simulink model "fundamental_component_calc"  (R2023a)
settings: Solver=VariableStepAuto  StartTime=0.0  StopTime=30  RelTol=1e-3
InitFcn:
  | Ts=100e-6;
libraries: powerlib_extras x2, simulink x1
settings Model: Creator=anony  LastModifiedBy=ym
settings SolverCC: AlgebraicLoopSolver=TrustRegion
settings OptimizationCC: ReuseModelBlockBuffer=off
settings DebuggingCC: UnconnectedInputMsg=warning  UnconnectedOutputMsg=warning  UnconnectedLineMsg=warning
settings ModelReferenceCC: EnableRefExpFcnMdlSchedulingChecks=on
settings RTWCC: DLArmComputeVersion=19.05

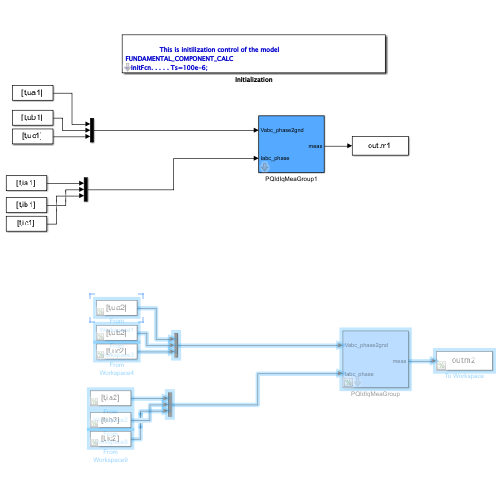
[thumbnail: Simulink's stored preview of the top-level diagram]
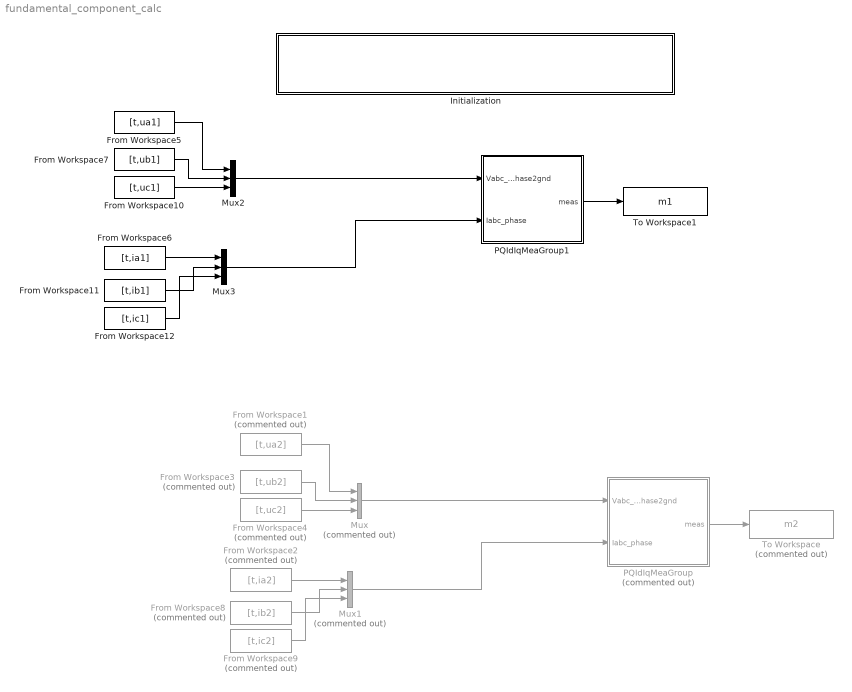
== system fundamental_component_calc ==
  From Workspace1 : FromWorkspace  Commented=on  VariableName=[t,ua2]
  From Workspace10 : FromWorkspace  VariableName=[t,uc1]
  From Workspace11 : FromWorkspace  VariableName=[t,ib1]
  From Workspace12 : FromWorkspace  VariableName=[t,ic1]
  From Workspace2 : FromWorkspace  Commented=on  VariableName=[t,ia2]
  From Workspace3 : FromWorkspace  Commented=on  VariableName=[t,ub2]
  From Workspace4 : FromWorkspace  Commented=on  VariableName=[t,uc2]
  From Workspace5 : FromWorkspace  VariableName=[t,ua1]
  From Workspace6 : FromWorkspace  VariableName=[t,ia1]
  From Workspace7 : FromWorkspace  VariableName=[t,ub1]
  From Workspace8 : FromWorkspace  Commented=on  VariableName=[t,ib2]
  From Workspace9 : FromWorkspace  Commented=on  VariableName=[t,ic2]
  Initialization : Subsystem  mask(Model Functions){InitFcnX=Ts=100e-6;, prel=off, posl=off, inif=on, strf=off}
      mask prompts: InitFcnX "Initialisation"; prel "Preload Function"; posl "PostLoad Function"; inif "InitFcn"; strf "StartFcn"
      mask init:
      | if prel==1
      | 	set_param(bdroot, 'PreLoadFcn', InitFcnX);
      | else
      | 	set_param(bdroot, 'PreLoadFcn', '');
      | end
      | if inif==1
      | 	set_param(bdroot, 'InitFcn', InitFcnX);
      | else
      | 	set_param(bdroot, 'InitFcn', '');
      | end
      | if strf==1
      | 	set_param(bdroot, 'StartFcn', InitFcnX);
      | else
      | 	set_param(bdroot, 'StartFcn', '');
      | end
      | if posl==1
      | 	set_param(bdroot, 'PostLoadFcn', InitFcnX);
      | else
      | 	set_param(bdroot, 'PostLoadFcn', '');
      | end
      | PLF = get_param(bdroot, 'PreLoadFcn');
      | IF = get_param(bdroot, 'InitFcn');
      | SF = get_param(bdroot, 'StartFcn');
      | 
      | 
      | pos = get_param(gcb, 'Position');
      | width = pos(3) - pos(1); height = pos(4) - pos(2);
      mask Display:
      | color('blue')
      | text(5, height*0.25, [ ...
      | upper(bdroot) '\n' ...
      | '- InitFcn. . . . . '  get_param(bdroot, 'InitFcn')  ...
      | ], ...
      | 'horizontalAlignment', 'left', 'verticalAlignment', 'middle') ;
      | text(60,height*0.6,'This is initilization control of the model');
  Mux : Mux  Commented=on  Inputs=3
  Mux1 : Mux  Commented=on  Inputs=3
  Mux2 : Mux  Inputs=3
  Mux3 : Mux  Inputs=3
  PQIdIqMeaGroup : Subsystem  Commented=on  mask{var_pnom=1.5e6, var_vline_rms=690, var_ts=Ts}
      mask prompts: var_pnom "Pnom"; var_vline_rms "Line voltage rms"; var_ts "Sample Time"
  PQIdIqMeaGroup1 : Subsystem  mask{var_pnom=1.5e6, var_vline_rms=690, var_ts=Ts}
      mask prompts: var_pnom "Pnom"; var_vline_rms "Line voltage rms"; var_ts "Sample Time"
  To Workspace : ToWorkspace  Commented=on  VariableName=m2  SaveFormat=Structure With Time  SampleTime=-1
  To Workspace1 : ToWorkspace  VariableName=m1  SaveFormat=Structure With Time  SampleTime=-1
  wires:
  Mux1/1 -> PQIdIqMeaGroup/2(Iabc_phase)
  Mux/1 -> PQIdIqMeaGroup/1(Vabc_phase2gnd)
  From Workspace4/1 -> Mux/3
  From Workspace3/1 -> Mux/2
  From Workspace1/1 -> Mux/1
  From Workspace9/1 -> Mux1/3
  From Workspace8/1 -> Mux1/2
  From Workspace2/1 -> Mux1/1
  PQIdIqMeaGroup/1(meas) -> To Workspace/1
  PQIdIqMeaGroup1/1(meas) -> To Workspace1/1
  From Workspace6/1 -> Mux3/1
  From Workspace11/1 -> Mux3/2
  From Workspace12/1 -> Mux3/3
  From Workspace5/1 -> Mux2/1
  From Workspace7/1 -> Mux2/2
  From Workspace10/1 -> Mux2/3
  Mux2/1 -> PQIdIqMeaGroup1/1(Vabc_phase2gnd)
  Mux3/1 -> PQIdIqMeaGroup1/2(Iabc_phase)

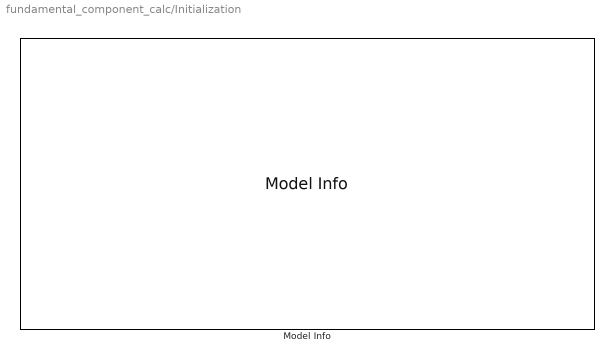
== system fundamental_component_calc/Initialization ==
  Model Info : simulink/Model-Wide Utilities/Model Info  Frame=on  DisplayStringWithTags=|  HorizontalTextAlignment=Center  LeftAlignmentValue=0.5
      | - Version <<<1.0 >>>
      | 
      | - Description :
      | %<Description>
      | 
      | - Created by :     %<Creator>
      | - Creation date : %<Created>
      | - Modified by :    %<ModifiedBy>
      | - Last modif. :   2012.12.11

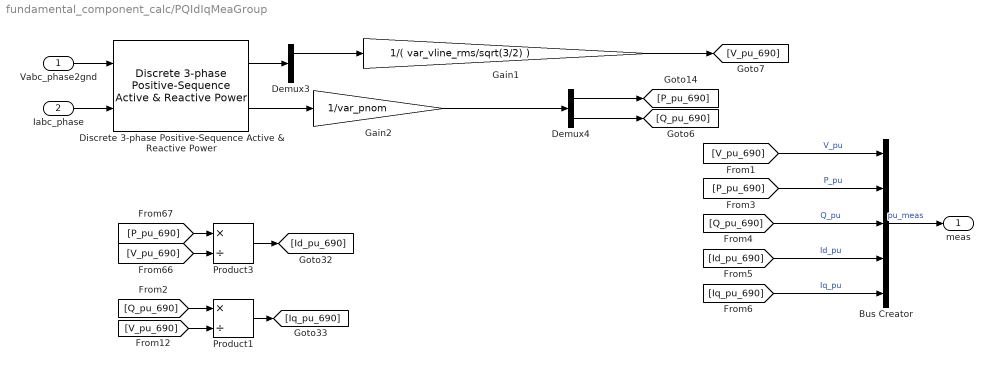
== system fundamental_component_calc/PQIdIqMeaGroup ==
  Vabc_phase2gnd : Inport
  Iabc_phase : Inport  Port=2
  Bus Creator : BusCreator  Inputs=5
  Demux3 : Demux  Outputs=2
  Demux4 : Demux  Outputs=2
  Discrete 3-phase Positive-Sequence Active & Reactive Power : powerlib_extras/Discrete Measurements/Discrete 3-phase  Positive-Sequence  Active & Reactive Power  Freq=50  Par_Vinit=[0 0]  Par_Iinit=[0 0]  Ts=Ts
  Gain1 : Gain  Gain=1/( var_vline_rms/sqrt(3/2) )
  Gain2 : Gain  Gain=1/var_pnom
  Product1 : Product  Inputs=*/  RndMeth=Zero
  Product3 : Product  Inputs=*/  RndMeth=Zero
  meas : Outport
  wires:
  Gain2/1 -> Demux4/1
  Gain1/1 -> [V_pu_690]
  Bus Creator/1 -> meas/1  "pu_meas"
  [Id_pu_690] -> Bus Creator/4  "Id_pu"
  [Iq_pu_690] -> Bus Creator/5  "Iq_pu"
  [Q_pu_690] -> Bus Creator/3  "Q_pu"
  [V_pu_690] -> Bus Creator/1  "V_pu"
  [P_pu_690] -> Bus Creator/2  "P_pu"
  [V_pu_690] -> Product3/2
  Product3/1 -> [Id_pu_690]
  [P_pu_690] -> Product3/1
  [V_pu_690] -> Product1/2
  [Q_pu_690] -> Product1/1
  Product1/1 -> [Iq_pu_690]
  Demux4/2 -> [Q_pu_690]
  Demux4/1 -> [P_pu_690]
  Discrete 3-phase Positive-Sequence Active & Reactive Power/2 -> Gain2/1
  Demux3/1 -> Gain1/1
  Discrete 3-phase Positive-Sequence Active & Reactive Power/1 -> Demux3/1
  Vabc_phase2gnd/1 -> Discrete 3-phase Positive-Sequence Active & Reactive Power/1
  Iabc_phase/1 -> Discrete 3-phase Positive-Sequence Active & Reactive Power/2

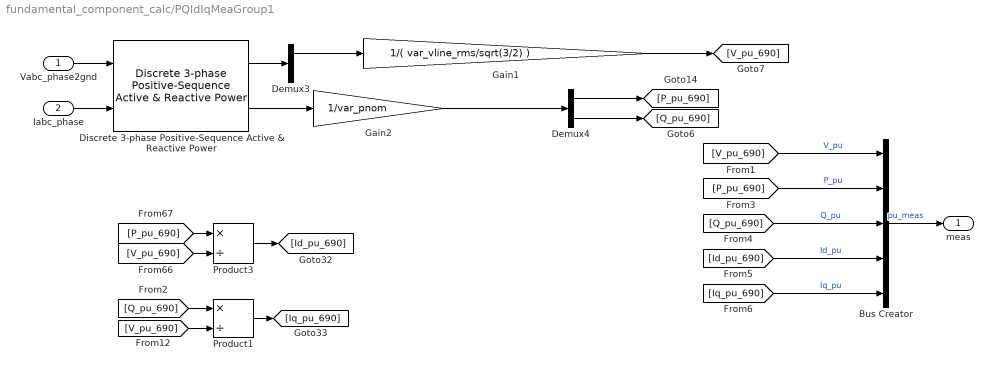
== system fundamental_component_calc/PQIdIqMeaGroup1 ==
  Vabc_phase2gnd : Inport
  Iabc_phase : Inport  Port=2
  Bus Creator : BusCreator  Inputs=5
  Demux3 : Demux  Outputs=2
  Demux4 : Demux  Outputs=2
  Discrete 3-phase Positive-Sequence Active & Reactive Power : powerlib_extras/Discrete Measurements/Discrete 3-phase  Positive-Sequence  Active & Reactive Power  Freq=50  Par_Vinit=[0 0]  Par_Iinit=[0 0]  Ts=Ts
  Gain1 : Gain  Gain=1/( var_vline_rms/sqrt(3/2) )
  Gain2 : Gain  Gain=1/var_pnom
  Product1 : Product  Inputs=*/  RndMeth=Zero
  Product3 : Product  Inputs=*/  RndMeth=Zero
  meas : Outport
  wires:
  Iabc_phase/1 -> Discrete 3-phase Positive-Sequence Active & Reactive Power/2
  Vabc_phase2gnd/1 -> Discrete 3-phase Positive-Sequence Active & Reactive Power/1
  Discrete 3-phase Positive-Sequence Active & Reactive Power/1 -> Demux3/1
  Demux3/1 -> Gain1/1
  Discrete 3-phase Positive-Sequence Active & Reactive Power/2 -> Gain2/1
  Demux4/1 -> [P_pu_690]
  Demux4/2 -> [Q_pu_690]
  Product1/1 -> [Iq_pu_690]
  [Q_pu_690] -> Product1/1
  [V_pu_690] -> Product1/2
  [P_pu_690] -> Product3/1
  Product3/1 -> [Id_pu_690]
  [V_pu_690] -> Product3/2
  [P_pu_690] -> Bus Creator/2  "P_pu"
  [V_pu_690] -> Bus Creator/1  "V_pu"
  [Q_pu_690] -> Bus Creator/3  "Q_pu"
  [Iq_pu_690] -> Bus Creator/5  "Iq_pu"
  [Id_pu_690] -> Bus Creator/4  "Id_pu"
  Bus Creator/1 -> meas/1  "pu_meas"
  Gain1/1 -> [V_pu_690]
  Gain2/1 -> Demux4/1
